simulink model "dynamics_2"  (R2020a)
settings: Solver=VariableStepAuto  StartTime=0.0  StopTime=10.0  RelTol=1e-3
values from neighbouring files (symbols this model uses):
  d = 1.1    [constants.m]    (also in navigation.m = 0.64; path_plan.m = 1851851851.85; test_2w_sensor.m = 0.64)
  J = 1000    [constants.m]
  Kb = 0.06    [constants.m]
  Kt = 11.43    [constants.m]
  l = 0.64    [constants.m]
  L = 0.125    [constants.m]    (also in ekf_func_test.m = 2.2; kin_model.m = 2.2; model.m = 2.2; navigation.m = 2.2)
  m = 810    [constants.m]    (also in path_plan.m = numel(x_s))
  r = 0.256    [constants.m]    (also in navigation.m; test_2w_sensor.m)
  R = 0.688    [constants.m]    (also in ekf_func_test.m = [1 0 0 0; kin_controller.m = @(theta) [cos(theta),sin(theta),0;-sin(theta),cos(theta),0;0; test.m = 10*[1 0 0 0; test_2w.m = 10*[1 0 0)
settings Model: Creator=anapi  LastModifiedBy=anapi

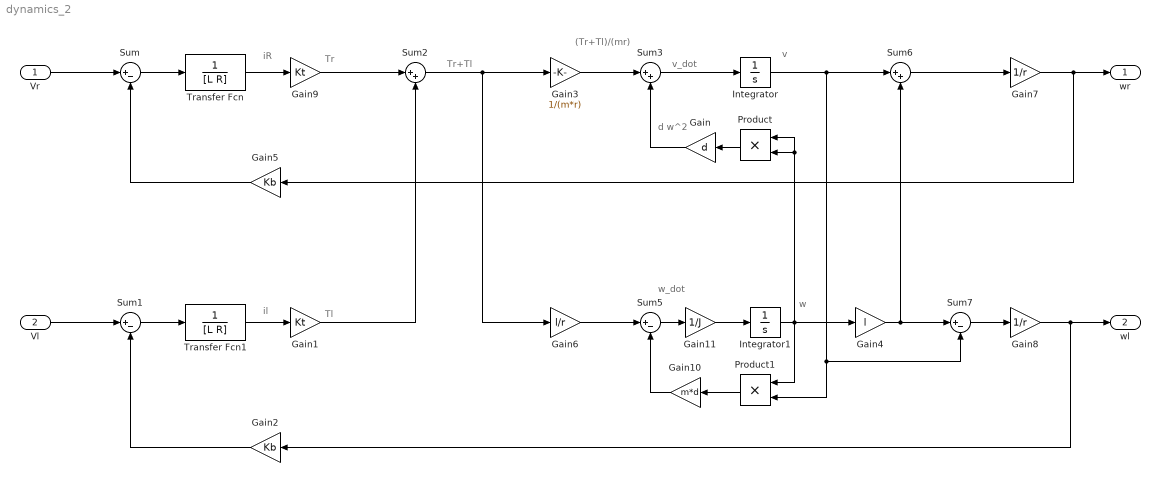
== system dynamics_2 ==
  note: d w^2
  note: (Tr+Tl)/(mr)
  note: v_dot
  note: iR
  note: Tr
  note: il
  note: Tl
  note: v
  note: w_dot
  note: w
  note: Tr+Tl
  Vr : Inport
  Vl : Inport  Port=2
  Gain : Gain  Gain=d
  Gain1 : Gain  Gain=Kt
  Gain10 : Gain  Gain=m*d
  Gain11 : Gain  Gain=1/J
  Gain2 : Gain  Gain=Kb
  Gain3 : Gain  Gain=1/(m*r)
  Gain4 : Gain  Gain=l
  Gain5 : Gain  Gain=Kb
  Gain6 : Gain  Gain=l/r
  Gain7 : Gain  Gain=1/r
  Gain8 : Gain  Gain=1/r
  Gain9 : Gain  Gain=Kt
  Integrator : Integrator
  Integrator1 : Integrator
  Product : Product
  Product1 : Product
  Sum{,1,5,7} (4 alike) : Sum  Inputs=|+-
  Sum2 : Sum  Inputs=|++
  Sum3 : Sum  Inputs=|++
  Sum6 : Sum  Inputs=|++
  Transfer Fcn : TransferFcn  Denominator=[L R]
  Transfer Fcn1 : TransferFcn  Denominator=[L R]
  wr : Outport
  wl : Outport  Port=2
  wires:
  Transfer Fcn/1 -> Gain9/1
  Sum/1 -> Transfer Fcn/1
  Vr/1 -> Sum/1
  Gain5/1 -> Sum/2
  Gain2/1 -> Sum1/2
  Vl/1 -> Sum1/1
  Gain1/1 -> Sum2/2
  Sum1/1 -> Transfer Fcn1/1
  Transfer Fcn1/1 -> Gain1/1
  Sum2/1 -> Gain3/1, Gain6/1
  Sum3/1 -> Integrator/1
  Gain6/1 -> Sum5/1
  Sum5/1 -> Gain11/1
  Integrator/1 -> Sum6/1, Product1/2, Sum7/2
  Integrator1/1 -> Product1/1, Product/1, Product/2, Gain4/1
  Gain4/1 -> Sum7/1, Sum6/2
  Sum6/1 -> Gain7/1
  Gain7/1 -> Gain5/1, wr/1
  Sum7/1 -> Gain8/1
  Gain8/1 -> Gain2/1, wl/1
  Gain9/1 -> Sum2/1
  Gain3/1 -> Sum3/1
  Product/1 -> Gain/1
  Gain/1 -> Sum3/2
  Product1/1 -> Gain10/1
  Gain10/1 -> Sum5/2
  Gain11/1 -> Integrator1/1
